simulink model "Henon_map"  (R2019b)
settings: Solver=VariableStepAuto  StartTime=0.0  StopTime=100  RelTol=1e-3  EnableMultiTasking=on
settings Model: Creator=Elena  LastModifiedBy=Elena

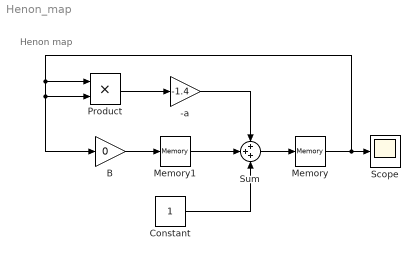
== system Henon_map ==
  note: Henon map
  "-a " : Gain  Gain=-1.4
  "B " : Gain  Gain=0
  Constant : Constant
  Memory : Memory
  Memory1 : Memory
  Product : Product
  Scope : Scope
  Sum : Sum  Inputs=+++
  wires:
  Constant/1 -> Sum/3
  Sum/1 -> Memory/1
  Memory/1 -> Product/1, "B "/1, Product/2, Scope/1
  "B "/1 -> Memory1/1
  Memory1/1 -> Sum/2
  Product/1 -> "-a "/1
  "-a "/1 -> Sum/1
